simulink subsystem "V_ideal"  (R2020a)
settings: Solver=VariableStepAuto  StartTime=0.0  StopTime=10.0  RelTol=1e-3
settings Model: Creator=Philip  LastModifiedBy=Philip

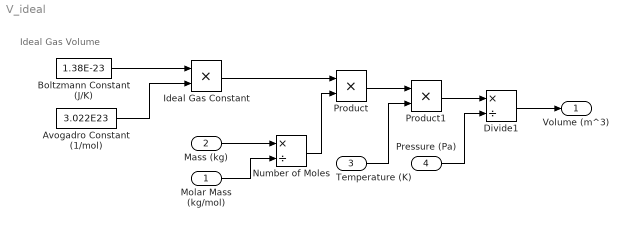
== system V_ideal ==
  note: Ideal Gas Volume
  Molar Mass (kg/mol) : Inport
  Mass (kg) : Inport  Port=2
  Temperature (K) : Inport  Port=3
  Pressure (Pa) : Inport  Port=4
  Avogadro Constant (1/mol) : Constant  Value=3.022E23
  Boltzmann Constant (J/K) : Constant  Value=1.38E-23
  Divide1 : Product  Inputs=*/
  Ideal Gas Constant : Product
  Number of Moles : Product  Inputs=*/
  Product : Product
  Product1 : Product
  Volume (m^3) : Outport
  wires:
  Mass (kg)/1 -> Number of Moles/1
  Molar Mass (kg/mol)/1 -> Number of Moles/2
  Divide1/1 -> Volume (m^3)/1
  Pressure (Pa)/1 -> Divide1/2
  Product1/1 -> Divide1/1
  Temperature (K)/1 -> Product1/2
  Product/1 -> Product1/1
  Number of Moles/1 -> Product/2
  Ideal Gas Constant/1 -> Product/1
  Boltzmann Constant (J/K)/1 -> Ideal Gas Constant/1
  Avogadro Constant (1/mol)/1 -> Ideal Gas Constant/2
